simulink library "SimpleFOCMini"  (R2024b)
settings: Solver=VariableStepAuto  StartTime=0.0  StopTime=10.0  RelTol=1e-3
settings Model: Creator=folke  LastModifiedBy=folke

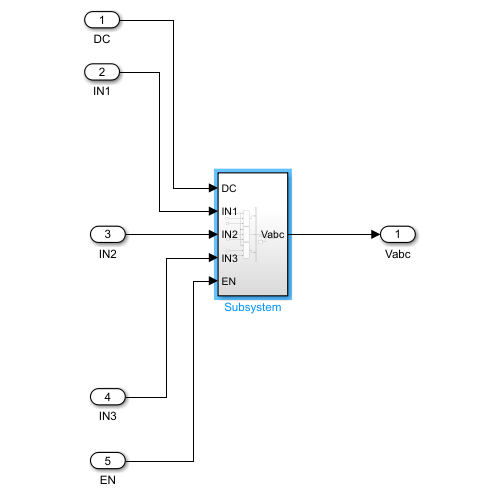
[thumbnail: Simulink's stored preview of the top-level diagram]
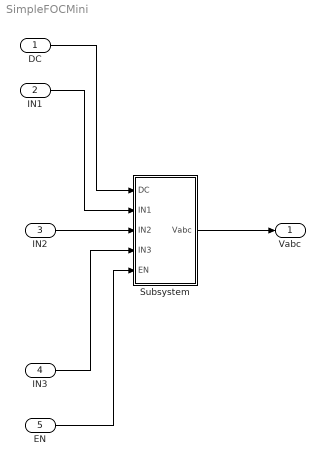
== system SimpleFOCMini ==
  DC : Inport
  IN1 : Inport  Port=2
  IN2 : Inport  Port=3
  IN3 : Inport  Port=4
  EN : Inport  Port=5
  Subsystem : Subsystem
  Vabc : Outport
  wires:
  DC/1 -> Subsystem/1(DC)
  IN1/1 -> Subsystem/2(IN1)
  IN2/1 -> Subsystem/3(IN2)
  IN3/1 -> Subsystem/4(IN3)
  EN/1 -> Subsystem/5(EN)
  Subsystem/1(Vabc) -> Vabc/1

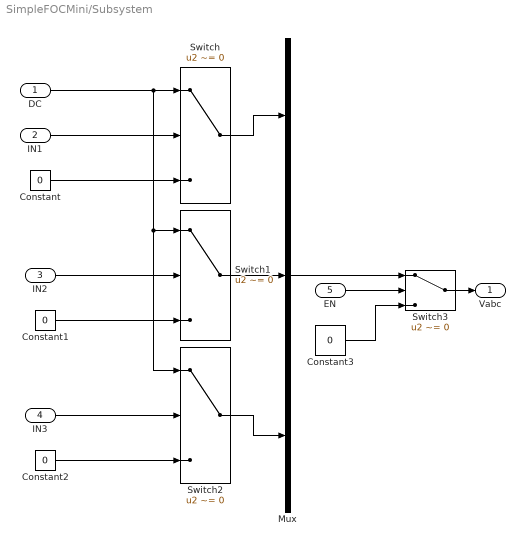
== system SimpleFOCMini/Subsystem ==
  DC : Inport
  IN1 : Inport  Port=2
  IN2 : Inport  Port=3
  IN3 : Inport  Port=4
  EN : Inport  Port=5
  Constant{,1..3} (4 alike) : Constant  Value=0
  Mux : Mux  Inputs=3
  Switch{,1..3} (4 alike) : Switch  Criteria=u2 ~= 0  SaturateOnIntegerOverflow=off  InputSameDT=off
  Vabc : Outport
  wires:
  Switch1/1 -> Mux/2
  Constant/1 -> Switch/3
  DC/1 -> Switch2/1, Switch1/1, Switch/1
  IN1/1 -> Switch/2
  IN2/1 -> Switch1/2
  Switch2/1 -> Mux/3
  IN3/1 -> Switch2/2
  EN/1 -> Switch3/2
  Switch3/1 -> Vabc/1
  Mux/1 -> Switch3/1
  Switch/1 -> Mux/1
  Constant1/1 -> Switch1/3
  Constant2/1 -> Switch2/3
  Constant3/1 -> Switch3/3
